simulink model "teach_learn"  (R2023a)
settings: Solver=ode2  StartTime=0.0  StopTime=inf  FixedStep=1/30  RelTol=1e-3  EnableMultiTasking=on
undefined symbols (not defined in the file): HIL, Host
libraries: quarc_library x8, simulink x1
settings Model: ExtModeTrigDuration=10000  Creator=msaravanan  LastModifiedBy=msaravanan
settings SolverCC: AlgebraicLoopSolver=TrustRegion  PositivePriorityOrder=on
settings DataIOCC: ReturnWorkspaceOutputs=off
settings DebuggingCC: UnconnectedInputMsg=warning  UnconnectedOutputMsg=warning  UnconnectedLineMsg=warning  ArithmeticOperatorsInVariantConditions=warning
settings ModelReferenceCC: EnableRefExpFcnMdlSchedulingChecks=on
settings SFSimCC: SimUseLocalCustomCode=off  CustomCodeUndefinedFunction=UseInterfaceOnly
settings RTWCC: Description=QUARC Win64 Target Using Toolchain  SystemTargetFile=quarc_win64.tlc  TemplateMakefile=quarc_default_tmf  RTWUseLocalCustomCode=off  Toolchain=QUARC win64 | nmake (64-bit Windows)  BuildConfiguration=Faster Runs
settings CodeAppCC: StateflowObjectComments=on
settings STFCustomTargetCC: SystemTargetFile=quarc_win64.tlc
settings GRTTargetCC: ParMdlRefBuildCompliant=off  CompOptLevelCompliant=off  CombineOutputUpdateFcns=off  MatFileLogging=off  CPPClassGenCompliant=off  GRTInterface=on  ExtMode=on  ExtModeMexFile=quarc_comm
settings ConfigComp: CovMetricSettings=dswe

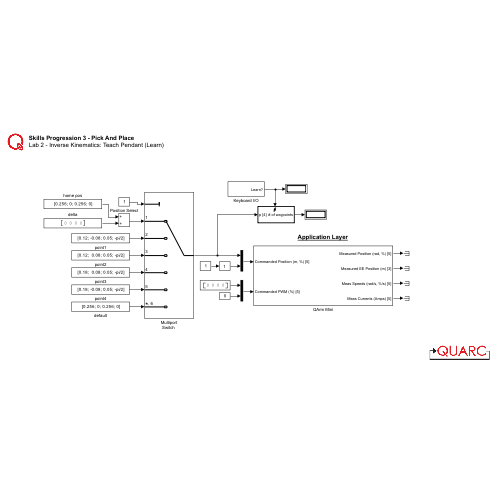
[thumbnail: Simulink's stored preview of the top-level diagram]
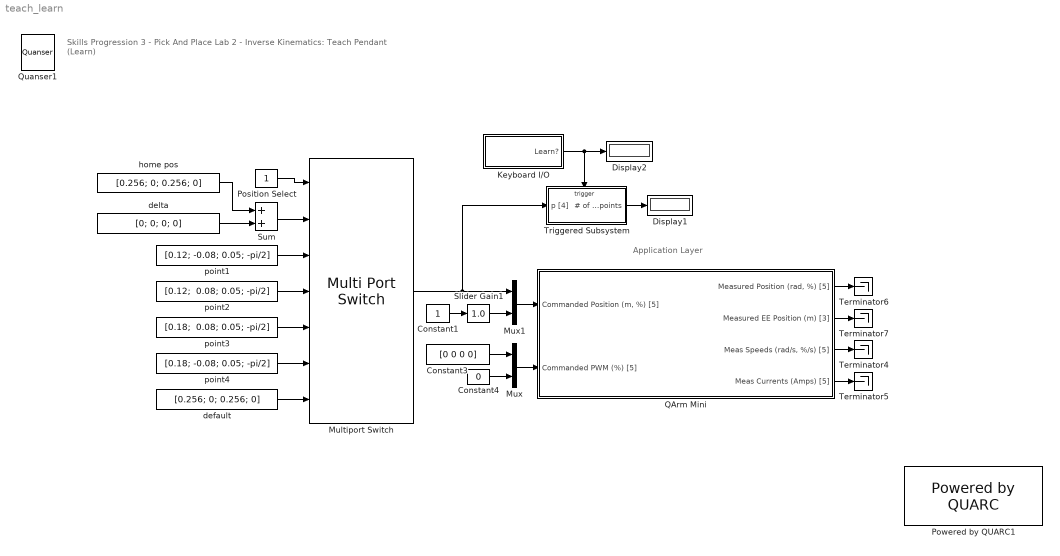
== system teach_learn ==
  note: Skills Progression 3 - Pick And Place
      | Lab 2 - Inverse Kinematics: Teach Pendant (Learn)
  note: Application Layer
  Constant1 : Constant
  Constant3 : Constant  Value=[0 0 0 0]
  Constant4 : Constant  Value=0
  Display1 : Display
  Display2 : Display
  Keyboard I/O : Subsystem
  "Multiport Switch " : MultiPortSwitch  Inputs=6  SaturateOnIntegerOverflow=off  InputSameDT=off
  Mux : Mux  Inputs=2
  Mux1 : Mux  Inputs=2
  Position Select : Constant
  Powered by QUARC1 : quarc_library/Logos/Powered by QUARC
  QArm Mini : Subsystem
  Quanser1 : quarc_library/Logos/Quanser
  Slider Gain1 : simulink/Math Operations/Slider Gain  gain=1.0  low=0  high=1
  Sum : Sum
  Terminator{4..7} (4 alike) : Terminator
  Triggered Subsystem : Subsystem  TreatAsAtomicUnit=on
  default : Constant  Value=[0.256; 0; 0.256; 0]
  delta : Constant  Value=[0; 0; 0; 0]
  home pos : Constant  Value=[0.256; 0; 0.256; 0]
  point1 : Constant  Value=[0.12; -0.08; 0.05; -pi/2]
  point2 : Constant  Value="[0.12;  0.08; 0.05; -pi/2]"
  point3 : Constant  Value="[0.18;  0.08; 0.05; -pi/2]"
  point4 : Constant  Value=[0.18; -0.08; 0.05; -pi/2]
  wires:
  QArm Mini/4(Meas Currents (Amps) [5]) -> Terminator5/1
  QArm Mini/1("Measured Position (rad, %) [5]") -> Terminator6/1
  Mux1/1 -> QArm Mini/1("Commanded Position (m, %) [5]")
  Constant3/1 -> Mux/1
  QArm Mini/3("Meas Speeds (rad/s, %/s) [5]") -> Terminator4/1
  Constant4/1 -> Mux/2
  Mux/1 -> QArm Mini/2(Commanded PWM (%) [5])
  Slider Gain1/1 -> Mux1/2
  Constant1/1 -> Slider Gain1/1
  Position Select/1 -> "Multiport Switch "/1
  point2/1 -> "Multiport Switch "/4
  point3/1 -> "Multiport Switch "/5
  point4/1 -> "Multiport Switch "/6
  point1/1 -> "Multiport Switch "/3
  "Multiport Switch "/1 -> Triggered Subsystem/1(p [4]), Mux1/1
  Triggered Subsystem/1(# of waypoints) -> Display1/1
  Keyboard I/O/1(Learn?) -> Triggered Subsystem/Trigger, Display2/1
  QArm Mini/2(Measured EE Position (m) [3]) -> Terminator7/1
  default/1 -> "Multiport Switch "/7
  Sum/1 -> "Multiport Switch "/2
  home pos/1 -> Sum/1
  delta/1 -> Sum/2

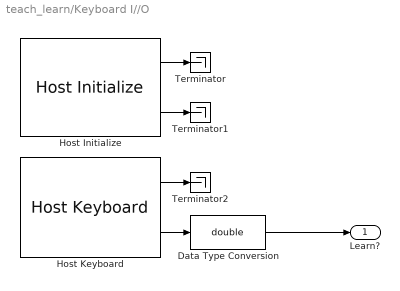
== system teach_learn/Keyboard I//O ==
  Data Type Conversion : DataTypeConversion  OutDataTypeStr=double  SaturateOnIntegerOverflow=off  RndMeth=Floor
  Host Initialize : quarc_library/Devices/Peripherals/Host/Host Initialize  object_name=Host-1  uri_source=Use external mode communications  uri=tcpip://localhost:18001  send_buffer_size=1000  receive_buffer_size=1000  thread_priority=0  run_client=on  use_window=off  window_position=[]  sample_time=qc_get_step_size  active=on
      settings: SourceProductName=QUARC Targets
  Host Keyboard : quarc_library/Devices/Peripherals/Host/Host Keyboard  object_name=Host-1  virtual_key=[32]  sample_time=qc_get_step_size  enabled=on  debug_mode=off
      settings: SourceProductName=QUARC Targets
  Terminator : Terminator
  Terminator1 : Terminator
  Terminator2 : Terminator
  Learn? : Outport
  wires:
  Host Initialize/1 -> Terminator/1
  Host Initialize/2 -> Terminator1/1
  Host Keyboard/1 -> Terminator2/1
  Host Keyboard/2 -> Data Type Conversion/1
  Data Type Conversion/1 -> Learn?/1

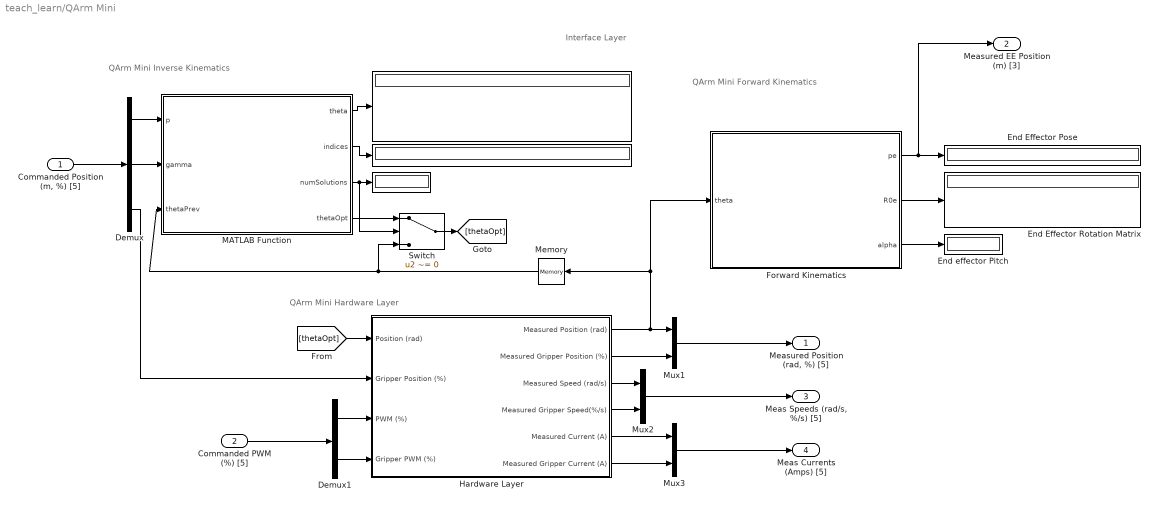
== system teach_learn/QArm Mini ==
  note: QArm Mini Inverse Kinematics
  note: QArm Mini Forward Kinematics
  note: Interface Layer
  note: QArm Mini Hardware Layer
  "Commanded Position (m, %) [5]" : Inport
  Commanded PWM (%) [5] : Inport  Port=2
  " " : Display
  "  " : Display
  "   " : Display
  Demux : Demux  Outputs=[3 1 1]
  Demux1 : Demux  Outputs=[4 1]
  End Effector Pose : Display
  End Effector Rotation Matrix : Display
  End effector Pitch : Display
  Forward Kinematics : MATLAB Function  TreatAsAtomicUnit=on
  Hardware Layer : Subsystem
  MATLAB Function : MATLAB Function  TreatAsAtomicUnit=on
  Memory : Memory  InitialCondition=[0; pi/2; -pi/2; pi/2]
  Mux1 : Mux  Inputs=2
  Mux2 : Mux  Inputs=2
  Mux3 : Mux  Inputs=2
  Switch : Switch  Criteria=u2 ~= 0  SaturateOnIntegerOverflow=off  InputSameDT=off
  "Measured Position (rad, %) [5]" : Outport
  Measured EE Position (m) [3] : Outport  Port=2
  "Meas Speeds (rad/s, %/s) [5]" : Outport  Port=3
  Meas Currents (Amps) [5] : Outport  Port=4
  wires:
  Hardware Layer/1(Measured Position (rad)) -> Forward Kinematics/1(theta), Memory/1, Mux1/1
  Forward Kinematics/2(R0e) -> End Effector Rotation Matrix/1
  Forward Kinematics/3(alpha) -> End effector Pitch/1
  Demux1/2 -> Hardware Layer/4(Gripper PWM (%))
  Hardware Layer/2(Measured Gripper Position (%)) -> Mux1/2
  Hardware Layer/3(Measured Speed (rad/s)) -> Mux2/1
  Hardware Layer/4(Measured Gripper Speed(%/s)) -> Mux2/2
  Hardware Layer/5(Measured Current (A)) -> Mux3/1
  Hardware Layer/6(Measured Gripper Current (A)) -> Mux3/2
  Mux3/1 -> Meas Currents (Amps) [5]/1
  Mux2/1 -> "Meas Speeds (rad/s, %/s) [5]"/1
  Mux1/1 -> "Measured Position (rad, %) [5]"/1
  "Commanded Position (m, %) [5]"/1 -> Demux/1
  Demux1/1 -> Hardware Layer/3(PWM (%))
  Commanded PWM (%) [5]/1 -> Demux1/1
  Forward Kinematics/1(pe) -> Measured EE Position (m) [3]/1, End Effector Pose/1
  Demux/1 -> MATLAB Function/1(p)
  Demux/2 -> MATLAB Function/2(gamma)
  Demux/3 -> Hardware Layer/2(Gripper Position (%))
  Memory/1 -> MATLAB Function/3(thetaPrev), Switch/3
  MATLAB Function/1(theta) -> "   "/1
  MATLAB Function/2(indices) -> "  "/1
  MATLAB Function/3(numSolutions) -> Switch/2, " "/1
  MATLAB Function/4(thetaOpt) -> Switch/1
  [thetaOpt] -> Hardware Layer/1(Position (rad))
  Switch/1 -> [thetaOpt]

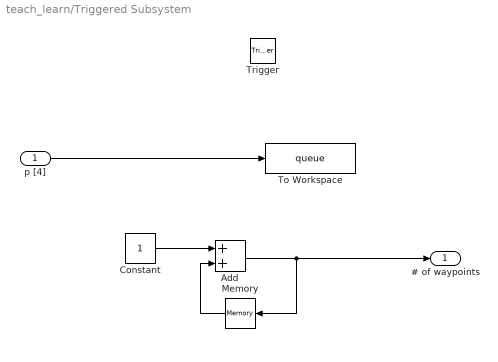
== system teach_learn/Triggered Subsystem ==
  p [4] : Inport
  Trigger : TriggerPort  VariantControl=(inherit)
  Add : Sum
  Constant : Constant
  Memory : Memory  InheritSampleTime=on
  To Workspace : ToWorkspace  VariableName=queue  SaveFormat=Structure  SampleTime=-1
  # of waypoints : Outport
  wires:
  p [4]/1 -> To Workspace/1
  Constant/1 -> Add/1
  Add/1 -> Memory/1, # of waypoints/1
  Memory/1 -> Add/2

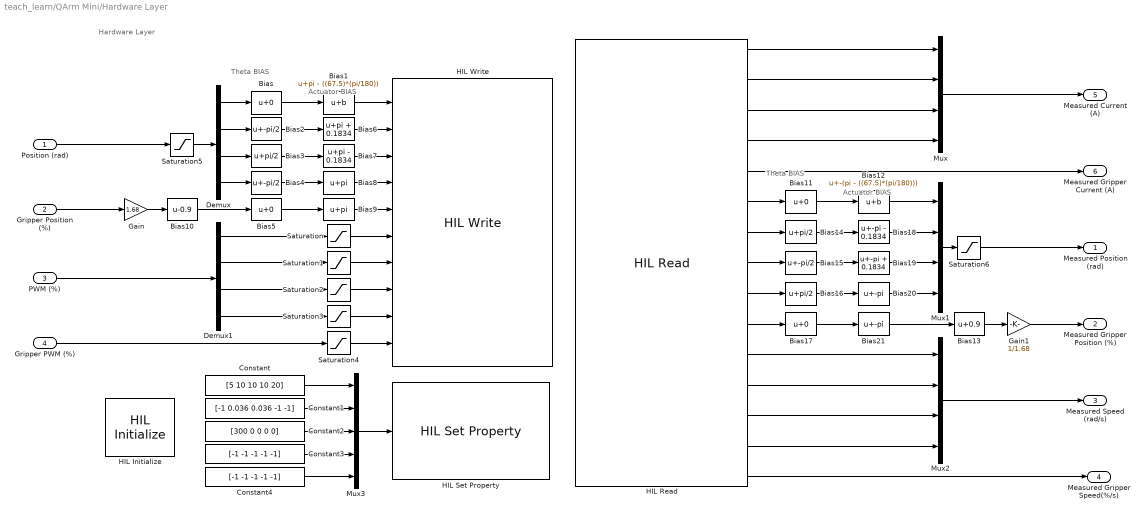
== system teach_learn/QArm Mini/Hardware Layer ==
  note: Hardware Layer
  note: Actuator BIAS
  note: Theta BIAS
  note: Actuator BIAS
  note: Theta BIAS
  Position (rad) : Inport
  Gripper Position (%) : Inport  Port=2
  PWM (%) : Inport  Port=3
  Gripper PWM (%) : Inport  Port=4
  Bias{,5,11,17} (4 alike) : Bias  SaturateOnIntegerOverflow=off
  Bias1 : Bias  Bias=pi - ((67.5)*(pi/180))  SaturateOnIntegerOverflow=off
  Bias10 : Bias  Bias=-0.9  SaturateOnIntegerOverflow=off
  Bias12 : Bias  Bias=-(pi - ((67.5)*(pi/180)))  SaturateOnIntegerOverflow=off
  Bias13 : Bias  Bias=0.9  SaturateOnIntegerOverflow=off
  Bias14 : Bias  Bias=pi/2  SaturateOnIntegerOverflow=off
  Bias15 : Bias  Bias=-pi/2  SaturateOnIntegerOverflow=off
  Bias16 : Bias  Bias=pi/2  SaturateOnIntegerOverflow=off
  Bias18 : Bias  Bias="-pi -  0.1834"  SaturateOnIntegerOverflow=off
  Bias19 : Bias  Bias="-pi +  0.1834"  SaturateOnIntegerOverflow=off
  Bias2 : Bias  Bias=-pi/2  SaturateOnIntegerOverflow=off
  Bias20 : Bias  Bias=-pi  SaturateOnIntegerOverflow=off
  Bias21 : Bias  Bias=-pi  SaturateOnIntegerOverflow=off
  Bias3 : Bias  Bias=pi/2  SaturateOnIntegerOverflow=off
  Bias4 : Bias  Bias=-pi/2  SaturateOnIntegerOverflow=off
  Bias6 : Bias  Bias=pi + 0.1834  SaturateOnIntegerOverflow=off
  Bias7 : Bias  Bias="pi -  0.1834"  SaturateOnIntegerOverflow=off
  Bias8 : Bias  Bias=pi  SaturateOnIntegerOverflow=off
  Bias9 : Bias  Bias=pi  SaturateOnIntegerOverflow=off
  Constant : Constant  Value=[5 10 10 10 20]
  Constant1 : Constant  Value=[-1 0.036 0.036 -1 -1]
  Constant2 : Constant  Value=[300 0 0 0 0]
  Constant3 : Constant  Value=[-1 -1 -1 -1 -1]
  Constant4 : Constant  Value=[-1 -1 -1 -1 -1]
  Demux : Demux
  Demux1 : Demux
  Gain : Gain  Gain=1.68
  Gain1 : Gain  Gain=1/1.68
  "HIL Initialize " : quarc_library/Data Acquisition/Generic/Configuration/HIL Initialize  object_name=HIL-1  board_type=qarm_mini  board_number=7  board_options=j0_mode=0;j1_mode=0;j2_mode=0;j3_mode=0;gripper_mode=0;j0_profile_velocity=6.2832;j0_profile_acceleration=6.2832;j1_profile_velocity=6.2832;j1_profile_acceleration=6.2832;j2_profile_velocity=6.2832;j2_profile_acceleration=6.2832;j3_profile_velocity=6.2832;j3_profile_acceleration=6.2832;gripper_profile_velocity=6.2832;gripper_profile_acceleration=6.2832;  exclusive=off  active=on  hardware_clocks=[]  clock_modes=[]  initial_clock_frequencies=[]  set_clock_params_at_start=off  set_clock_params_at_switch_in=off  set_clock_frequencies_at_start=off  set_clock_frequencies_at_switch_in=off  analog_input_channels=[0:4]  analog_input_configurations=[]  analog_input_maximums=[100 3.21 3.21 3.21 100]  analog_input_minimums=[-100 -3.21 -3.21 -3.21 -100]  set_analog_input_params_at_start=off  set_analog_input_params_at_switch_in=off  analog_output_channels=[]  analog_output_maximums=[]  analog_output_minimums=[]  initial_analog_outputs=[]  final_analog_outputs=[]  watchdog_analog_outputs=[]  set_analog_output_params_at_start=off  set_analog_output_params_at_switch_in=off  set_analog_outputs_at_start=off  set_analog_outputs_at_switch_in=off  set_analog_outputs_at_terminate=off  set_analog_outputs_at_switch_out=off  set_analog_outputs_on_watchdog=off  digital_input_channels=[]  digital_output_channels=[]  digital_output_configuration=[]  initial_digital_outputs=[]  final_digital_outputs=[]  watchdog_digital_outputs=[]  set_digital_output_params_at_start=off  set_digital_output_params_at_switch_in=off  set_digital_outputs_at_start=off  set_digital_outputs_at_switch_in=off  set_digital_outputs_at_terminate=off  set_digital_outputs_at_switch_out=off  set_digital_outputs_on_watchdog=off  encoder_channels=[]  quadrature=[]  encoder_filter_frequency=[]  initial_encoder_counts=[]  set_encoder_params_at_start=off  set_encoder_params_at_switch_in=off  set_encoder_counts_at_start=off  set_encoder_counts_at_switch_in=off  pwm_channels=[]  pwm_modes=[]  pwm_frequency=[]  pwm_configuration=[]  pwm_alignment=[]  pwm_polarity=[]  pwm_leading_deadband=[]  pwm_trailing_deadband=[]  initial_pwm_outputs=[]  final_pwm_outputs=[]  watchdog_pwm_outputs=[]  set_pwm_params_at_start=off  set_pwm_params_at_switch_in=off  set_pwm_outputs_at_start=off  set_pwm_outputs_at_switch_in=off  set_pwm_outputs_at_terminate=off  set_pwm_outputs_at_switch_out=off  set_pwm_outputs_on_watchdog=off  other_output_channels=[]  initial_other_outputs=[]  final_other_outputs=[]  watchdog_other_outputs=[]  set_other_outputs_at_start=off  set_other_outputs_at_switch_in=off  set_other_outputs_at_terminate=off  set_other_outputs_at_switch_out=off  set_other_outputs_on_watchdog=off
  HIL Read : quarc_library/Data Acquisition/Generic/Immediate I//O/HIL Read  object_name=HIL-1  analog_channels=[0:4]  encoder_channels=[]  digital_channels=[]  other_channels=[1000:1004 3000:3004]  sample_time=qc_get_step_size  active=on  vector_output=off  data_type_mode=Inherit via back propagation  encoder_data_type=double  digital_data_type=boolean
  HIL Set Property : quarc_library/Data Acquisition/Generic/Configuration/HIL Set Property  object_name=HIL-1  property_type=2  property_codes=[128:152]  property_source=2  property_value_num=0  set_at_start=on  sample_time=-1  active=off
      settings: AttributesFormatString=(%<object_name>)  SourceProductName=QUARC Targets
  HIL Write : quarc_library/Data Acquisition/Generic/Immediate I//O/HIL Write  object_name=HIL-1  analog_channels=[]  pwm_channels=[]  digital_channels=[]  other_channels=[1000:1004 11000:11004]  sample_time=-1  active=off  vector_input=off
  Mux : Mux
  Mux1 : Mux
  Mux2 : Mux
  Mux3 : Mux  Inputs=5
  Saturation{,1..4} (5 alike) : Saturate
  Saturation5 : Saturate  UpperLimit=[5*pi/4, pi, 0, 3*pi/4]'  LowerLimit=[-pi/2. 0, -3*pi/4, 0]'
  Saturation6 : Saturate  UpperLimit=[5*pi/4, pi, 0, 3*pi/4]'  LowerLimit=[-pi/2. 0, -3*pi/4, 0]'
  Measured Position (rad) : Outport
  Measured Gripper Position (%) : Outport  Port=2
  Measured Speed (rad/s) : Outport  Port=3
  Measured Gripper Speed(%/s) : Outport  Port=4
  Measured Current (A) : Outport  Port=5
  Measured Gripper Current (A) : Outport  Port=6
  wires:
  Position (rad)/1 -> Saturation5/1
  Demux/2 -> Bias2/1
  Demux/3 -> Bias3/1
  Demux/4 -> Bias4/1
  Bias/1 -> Bias1/1
  Bias1/1 -> HIL Write/1
  Bias2/1 -> Bias6/1
  Bias6/1 -> HIL Write/2
  Bias3/1 -> Bias7/1
  Bias7/1 -> HIL Write/3
  Bias4/1 -> Bias8/1
  Bias8/1 -> HIL Write/4
  Bias5/1 -> Bias9/1
  Bias9/1 -> HIL Write/5
  Gain/1 -> Bias10/1
  PWM (%)/1 -> Demux1/1
  Gripper PWM (%)/1 -> Saturation4/1
  Saturation/1 -> HIL Write/6
  Saturation1/1 -> HIL Write/7
  Saturation2/1 -> HIL Write/8
  Saturation3/1 -> HIL Write/9
  Saturation4/1 -> HIL Write/10
  HIL Read/1 -> Mux/1
  HIL Read/2 -> Mux/2
  HIL Read/3 -> Mux/3
  HIL Read/4 -> Mux/4
  Mux/1 -> Measured Current (A)/1
  HIL Read/5 -> Measured Gripper Current (A)/1
  Bias14/1 -> Bias18/1
  Bias15/1 -> Bias19/1
  Bias17/1 -> Bias21/1
  Bias11/1 -> Bias12/1
  Bias16/1 -> Bias20/1
  HIL Read/6 -> Bias11/1
  HIL Read/7 -> Bias14/1
  HIL Read/8 -> Bias15/1
  HIL Read/9 -> Bias16/1
  HIL Read/10 -> Bias17/1
  Bias21/1 -> Bias13/1
  Bias13/1 -> Gain1/1
  Gain1/1 -> Measured Gripper Position (%)/1
  Mux1/1 -> Saturation6/1
  HIL Read/11 -> Mux2/1
  HIL Read/12 -> Mux2/2
  HIL Read/13 -> Mux2/3
  HIL Read/14 -> Mux2/4
  Mux2/1 -> Measured Speed (rad/s)/1
  HIL Read/15 -> Measured Gripper Speed(%/s)/1
  Constant/1 -> Mux3/1
  Constant1/1 -> Mux3/2
  Constant2/1 -> Mux3/3
  Constant3/1 -> Mux3/4
  Constant4/1 -> Mux3/5
  Mux3/1 -> HIL Set Property/1
  Bias12/1 -> Mux1/1
  Bias18/1 -> Mux1/2
  Bias19/1 -> Mux1/3
  Bias20/1 -> Mux1/4
  Demux1/1 -> Saturation/1
  Demux1/2 -> Saturation1/1
  Demux1/3 -> Saturation2/1
  Demux1/4 -> Saturation3/1
  Demux/1 -> Bias/1
  Saturation5/1 -> Demux/1
  Saturation6/1 -> Measured Position (rad)/1
  Gripper Position (%)/1 -> Gain/1
  Bias10/1 -> Bias5/1

== matlab function teach_learn/QArm Mini/MATLAB Function ==
  data: p input; theta output; gamma input; thetaPrev input; indices output; numSolutions output; thetaOpt output
function [theta, indices, numSolutions, thetaOpt] = qArmMiniInverseKinematics(p, gamma, thetaPrev)

%% QUANSER_ARM_IPK
% v 1.2 - 2nd December 2022

% REFERENCE: 
% Chapter 4. Inverse Kinematics
% Robot Dynamics and Control 
% Spong, Vidyasagar
% 1989

% INPUTS:
% p         : end-effector position vector expressed in base frame {0}
% gamma     : wrist rotation angle gamma
% thetaPrev : previous joint positions

% OUTPUTS:
% thetaOpt      : Best solution depending on theta_prev
% theta         : Upto 4 solutions, each col is a solution.
% numSolutions  : number of valid solutions based on joint limits
% indices       : indices of which solutions are valid
%                        0 - not valid 
%                        1 - valid solution
%                        2 - optimal solution
%% Manipulator parameters:
L1 = 0.1300;
L2 = 0.1240;
L3 = 0.0230;
L4 = 0.1240;
L5 = 0.1320;

%% Alternate parameters
l1 = L1;
l2 = sqrt(L2^2 + L3^2);
l3 = L4;
l4 = L5;

%% Initialization
theta         = zeros(4, 4);
thetaOpt      = zeros(4, 1);
d1_flag       = 0;
d2_flag       = 0;
indices       = zeros(4,1);
indexModifier = 0;
%% Joint angle 2 and 3: 
% Standard paramters. D has 2 possible values, and correspondingly F
% has two values as well. 
A = l2;
B = l3;
D1 =  sqrt(p(1)^2 + p(2)^2) - l4*cos(gamma);
D2 = -sqrt(p(1)^2 + p(2)^2) - l4*cos(gamma);
H =  p(3) - l1 - l4*sin(gamma);
F1 = (D1^2 + H^2 - A^2 - B^2)/(2*A);
F2 = (D2^2 + H^2 - A^2 - B^2)/(2*A);

% Evaluate the total number of solutions. The solution for joint 3
% requires us to calculate the square root of B^2 - F^2. For this, the
% F1 and F2 terms cannot be larger than B in magnitude. Determining
% which ones violate this condition will help us narrow down solutions
% from 4 to 2 to 0. Note that this check does not eliminate solutions that
% are not feasible due to joint limits, neither does it check for the
% closest solution to theta_prev. That happens later.
if B^2 < F1^2 && B^2 < F2^2
    % Both conditions are violated, so no solutions exist
    numSolutions = 0;
    return
elseif B^2 < F1^2 && B^2 >= F2^2
    % F1 is a problem, F2 is not, 2 solutions exist
    numSolutions = 2;
    d2_flag = 1;
elseif B^2 < F2^2 && B^2 >= F1^2
    % F2 is a problem, F1 is not, 2 solutions exist
    numSolutions = 2;
    d1_flag = 1;
else
    % 4 solutions exist theoretically!
    numSolutions = 4;
    d1_flag = 1;
    d2_flag = 1;
end

% Now that the d1_flag and d2_flag are raised to highlight which conditions
% were not violated, we can use them to evaluate theta(3) and theta(2).
if d1_flag
    % there are 2 possible values for theta(3) based on the + or - sqrt.
    theta(3,1) = 2*atan2(  sqrt(B^2 - F1^2) , B + F1 );
    theta(3,2) = 2*atan2( -sqrt(B^2 - F1^2) , B + F1 );

    % solve the 2 possible theta(2) values based on the theta(3) ones
    % that were just found.

    % theta(2,1) from theta(3,1)
    M = B*cos(theta(3,1));
    N = B*sin(theta(3,1));
    cos_term = (D1*A + D1*M + H*N)/((A + M)^2 + N^2);
    sin_term = (H*A + H*M - D1*N)/((A + M)^2 + N^2);
    theta(2,1) = atan2(sin_term, cos_term);

    % theta(2,2) from theta(3,2)
    M = B*cos(theta(3,2));
    N = B*sin(theta(3,2));
    cos_term = (D1*A + D1*M + H*N)/((A + M)^2 + N^2);
    sin_term = (H*A + H*M - D1*N)/((A + M)^2 + N^2);
    theta(2,2) = atan2(sin_term, cos_term);
    
    % Find the two corresponding theta(1) solutions using theta(2) and
    % theta(3)
    theta(1,1) = atan2( p(2)/( l2 * cos( theta(2,1) ) + l3 * cos( theta(2,1) + theta(3,1) ) + l4 * cos( gamma ) ) , p(1)/(  l2 * cos( theta(2,1) ) + l3 * cos( theta(2,1) + theta(3,1) ) + l4 * cos( gamma ) ) );
    theta(1,2) = atan2( p(2)/( l2 * cos( theta(2,2) ) + l3 * cos( theta(2,2) + theta(3,2) ) + l4 * cos( gamma ) ) , p(1)/(  l2 * cos( theta(2,2) ) + l3 * cos( theta(2,2) + theta(3,2) ) + l4 * cos( gamma ) ) );
end

if d2_flag 
    % check if the 2 solutions below are solutions (1 & 2) or (3 & 4) based
    % on whether numSolutions was set to 4 or not. If you are here, it was
    % definitely 4 or 2.
    if numSolutions == 4
        indexModifier = 2; % will ensure that solutions 
                           % are saved to locations with 
                           % a 2 offset
    else
        indexModifier = 0;
    end
    
    % there are 2 possible values for theta(3) based on the + or - sqrt.
    theta(3,1+indexModifier) = 2*atan2(  sqrt(B^2 - F2^2) , B + F2 );
    theta(3,2+indexModifier) = 2*atan2( -sqrt(B^2 - F2^2) , B + F2 );
    
    % solve the 2 possible theta(2) values based on the theta(3) ones
    % that were just found.

    % theta(2,1) from theta(3,1)
    M = B*cos(theta(3,1+indexModifier));
    N = B*sin(theta(3,1+indexModifier));
    cos_term = (D2*A + D2*M + H*N)/((A + M)^2 + N^2);
    sin_term = (H*A + H*M - D2*N)/((A + M)^2 + N^2);
    theta(2,1+indexModifier) = atan2(sin_term, cos_term);

    % theta(2,2) from theta(3,2)
    M = B*cos(theta(3,2+indexModifier));
    N = B*sin(theta(3,2+indexModifier));
    cos_term = (D2*A + D2*M + H*N)/((A + M)^2 + N^2);
    sin_term = (H*A + H*M - D2*N)/((A + M)^2 + N^2);
    theta(2,2+indexModifier) = atan2(sin_term, cos_term);

    % Find the two corresponding theta(1) solutions using theta(2) and
    % theta(3)
    theta(1,1+indexModifier) = atan2( p(2)/( l2 * cos( theta(2,1+indexModifier) ) + l3 * cos( theta(2,1+indexModifier) + theta(3,1+indexModifier) ) + l4 * cos( gamma ) ) , p(1)/(  l2 * cos( theta(2,1+indexModifier) ) + l3 * cos( theta(2,1+indexModifier) + theta(3,1+indexModifier) ) + l4 * cos( gamma ) ) );
    theta(1,2+indexModifier) = atan2( p(2)/( l2 * cos( theta(2,2+indexModifier) ) + l3 * cos( theta(2,2+indexModifier) + theta(3,2+indexModifier) ) + l4 * cos( gamma ) ) , p(1)/(  l2 * cos( theta(2,2+indexModifier) ) + l3 * cos( theta(2,2+indexModifier) + theta(3,2+indexModifier) ) + l4 * cos( gamma ) ) );
end

%% Joint angle 4:
if d1_flag
    theta(4,1) = gamma + pi/2 - theta(2, 1) - theta(3, 1);
    theta(4,2) = gamma + pi/2 - theta(2, 2) - theta(3, 2);
    indices(1,1) = 1;
    indices(2,1) = 1;
end
if d2_flag
    theta(4,1+indexModifier) = gamma + pi/2 - theta(2, 1+indexModifier) - theta(3, 1+indexModifier);
    theta(4,2+indexModifier) = gamma + pi/2 - theta(2, 2+indexModifier) - theta(3, 2+indexModifier);
    indices(3,1) = 1;
    indices(4,1) = 1;
end
%% Joint checks and final modifications

% saturate theta values from -pi to pi
% theta = mod(theta + pi, 2*pi) - pi;

% indices = [ones(numSolutions, 1), zeros(4-numSolutions, 1)];
numSolutionsMod = 0;

% find which solutions are valid based on joint limits
for i = 1:numSolutions
    if check_joint_limits(theta(:,i))
        indices(i) = 0;
        numSolutionsMod = numSolutionsMod - 1;
    end	
end
numSolutions = numSolutions + numSolutionsMod;

if numSolutions == 1
    for i = 1:4
        if (indices(i) > 0)
            indices(i) = 2;
            thetaOpt = theta(:,i);
        end
    end
end

if numSolutions > 1
    % % find the solution from thetas that is closest to thetaPrev
    % closestSolution = theta(:,1);
    % mark = 1;
    % for i = 2:4
    %     if indices(i)
    %         if norm(theta(:,i) - thetaPrev, 2) < norm(closestSolution - thetaPrev, 2)
    %             closestSolution = theta(:,i);
    %             mark = i;
    %         end
    %     end
    % end
    mark = 0;
    mark = check_closest_solution(theta,thetaPrev, indices);
    indices(mark) = 2;
    thetaOpt = theta(:,mark);
end

end

function flag = check_joint_limits(theta)
% flag is 0 by default (no issues)
% if any of the theta values are not in the correct joint limits, raise the
% flag.
flag = 0;
    % if (   theta(1) > -pi/2       || theta(1) < 5*pi/4 ...
    %     || theta(2) > -pi/2       || theta(2) < pi/2 ...
    %     || theta(3) > -pi/4       || theta(3) < pi/2 ...
    %     || theta(4) > -pi/2       || theta(4) < pi/4)

    if (   theta(1) > 225*pi/180 || theta(1) < -90*pi/180 ...
        || theta(2) > 180*pi/180 || theta(2) <    0*pi/180 ...
        || theta(3) >   0*pi/180 || theta(3) < -135*pi/180 ...
        || theta(4) > 157.5*pi/180 || theta(4) < 0*pi/180 )

        flag = 1;
    end
end

function mark = check_closest_solution(theta, thetaPrev, indices)
    closestSolution = zeros(4, 4);
    mark = 0;
    % Find the first valid solution to check against
    for i = 1:4
        if (indices(i) > 0)
            %mark = i
            closestSolution = theta(:,i);
            break;
        end
    end

    for i = 1:4
        if indices(i)
            if norm(theta(:,i) - thetaPrev, 2) < norm(closestSolution - thetaPrev, 2)
                closestSolution = theta(:,i);
                mark = i;
            end
        end
    end

end

== matlab function teach_learn/QArm Mini/Forward Kinematics ==
  data: theta input; pe output; R0e output; alpha output
function [pe, R0e, alpha] = qArmMiniForwardKinematics(theta)

%% QARM_MINI_FPK
% v 1.0 - 30th March 2025

% REFERENCE: 
% Chapter 3. Forward Kinematics
% Robot Dynamics and Control 
% Spong, Vidyasagar
% 1989

% INPUTS:
% theta   : Alternate joint angles vector 4 x 1

% OUTPUTS:
% pe      : End-effector frame {e} position vector expressed in base frame {0}
% R0e     : rotation matrix from end-effector frame {e} to base frame {0}

%% Manipulator parameters:
L1 = 0.1300;
L2 = 0.1240;
L3 = 0.0230;
L4 = 0.1240;
L5 = 0.1320;

%% Alternate parameters
l1 = L1;
l2 = sqrt(L2^2 + L3^2);
l3 = L4;
l4 = L5;

%% Transformation matrices for all frames:

% T{i-1}{i} = quanser_arm_DH(  a, alpha,  d,     theta );
        T01 = quanser_arm_DH(  0,  pi/2, l1,  theta(1) );
        T12 = quanser_arm_DH( l2,     0,  0,  theta(2) );
        T23 = quanser_arm_DH( l3,     0,  0,  theta(3) );
        T34 = quanser_arm_DH(  0,  pi/2,  0,  theta(4) );
        T4e = quanser_arm_DH(  0,     0, l4,         0 );
        
        T02 = T01*T12;
        T03 = T02*T23;
        T04 = T03*T34;
        T0e = T04*T4e;
        
%% Position of end-effector Transformation

% Extract the Position vector 
p1   = T01(1:3,4);
p2   = T02(1:3,4);
p3   = T03(1:3,4);
p4   = T04(1:3,4);
pe   = T0e(1:3,4);

% Extract the Rotation matrix
R01 = T01(1:3,1:3);
R02 = T02(1:3,1:3);
R03 = T03(1:3,1:3);
R04 = T04(1:3,1:3);
R0e = T0e(1:3,1:3);
alpha = theta(2) + theta(3) + theta(4) - pi/2;
end

function T = quanser_arm_DH(a,alpha,d,theta)

%% QUANSER_ARM_DH
% v 1.0 - 26th March 2019

% REFERENCE: 
% Chapter 3. Forward and Inverse Kinematics
% Robot Modeling and Control 
% Spong, Hutchinson, Vidyasagar
% 2006

% INPUTS:
% a       :   translation  : along : x_{i}   : from : z_{i-1} : to : z_{i}
% alpha   :      rotation  : about : x_{i}   : from : z_{i-1} : to : z_{i}
% d       :   translation  : along : z_{i-1} : from : x_{i-1} : to : x_{i}
% theta   :      rotation  : about : z_{i-1} : from : x_{i-1} : to : x_{i}
% NOTE: Standard DH Parameters

% OUTPUTS:
% T       : transformation                   : from :     {i} : to : {i-1}

%%
% Rotation Transformation about z axis by theta
T_R_z = [cos(theta) -sin(theta) 0 0;
         sin(theta)  cos(theta) 0 0;
                  0           0 1 0;
                  0           0 0 1];
     
% Translation Transformation along z axis by d
T_T_z = [1 0 0 0;
         0 1 0 0;
         0 0 1 d;
         0 0 0 1];

% Translation Transformation along x axis by a
T_T_x = [1 0 0 a;
         0 1 0 0;
         0 0 1 0;
         0 0 0 1];

% Rotation Transformation about x axis by alpha
T_R_x = [1          0           0 0;
         0 cos(alpha) -sin(alpha) 0;
         0 sin(alpha)  cos(alpha) 0;
         0          0           0 1];

% For a transformation FROM frame {i} TO frame {i-1}: A
T = T_R_z*T_T_z*T_T_x*T_R_x;

end
